simulink library "TorqueCommand"  (R2025a)
settings: Solver=VariableStepAuto  StartTime=0.0  StopTime=10.0  RelTol=1e-3
values from neighbouring files (symbols this model uses):
  RegenEnable : value not decoded    [TorqueCommand.sldd]
  TCEnable : value not decoded    [TorqueCommand.sldd]
undefined symbols (not defined in the file or in its folder): DiscIntNeverNeededParam, dt, raptor_xcp_function, TorqueKiLowerSat, TorqueKiUpperSat
libraries: Raptor_lib x56, Utilities x14, simulink x7, $bdroot x5
(part 1 of 2)
settings Model: Creator=serga  LastModifiedBy=hyuga

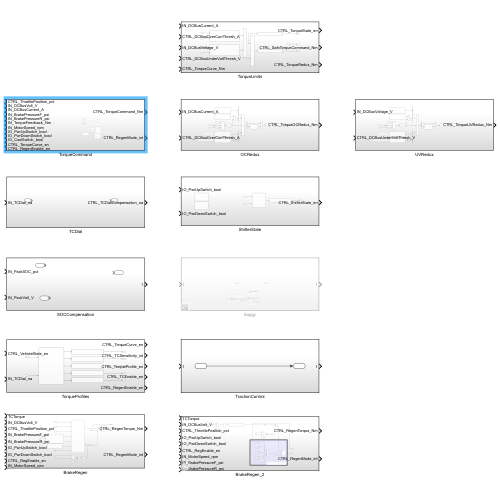
[thumbnail: Simulink's stored preview of the top-level diagram]
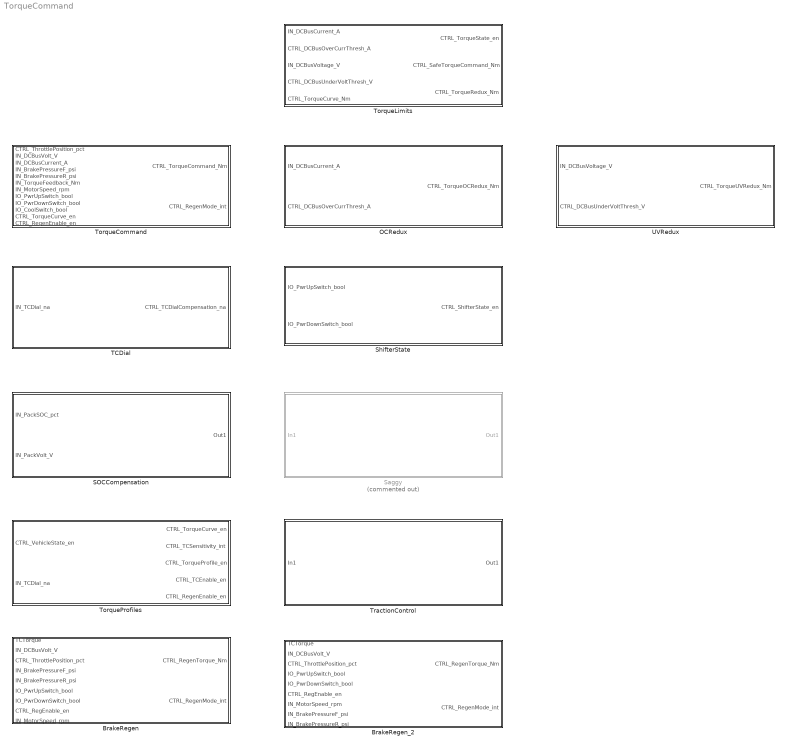
== system TorqueCommand ==
  BrakeRegen : Subsystem
  BrakeRegen_2 : Subsystem  AncestorBlock=TorqueCommand/BrakeRegen
  OCRedux : Subsystem
  SOCCompensation : Subsystem
  Saggy : Subsystem  Commented=on
  ShifterState : Subsystem
  TCDial : Subsystem
  TorqueCommand : Subsystem
  TorqueLimits : Subsystem
  TorqueProfiles : Subsystem
  TractionControl : Subsystem
  UVRedux : Subsystem

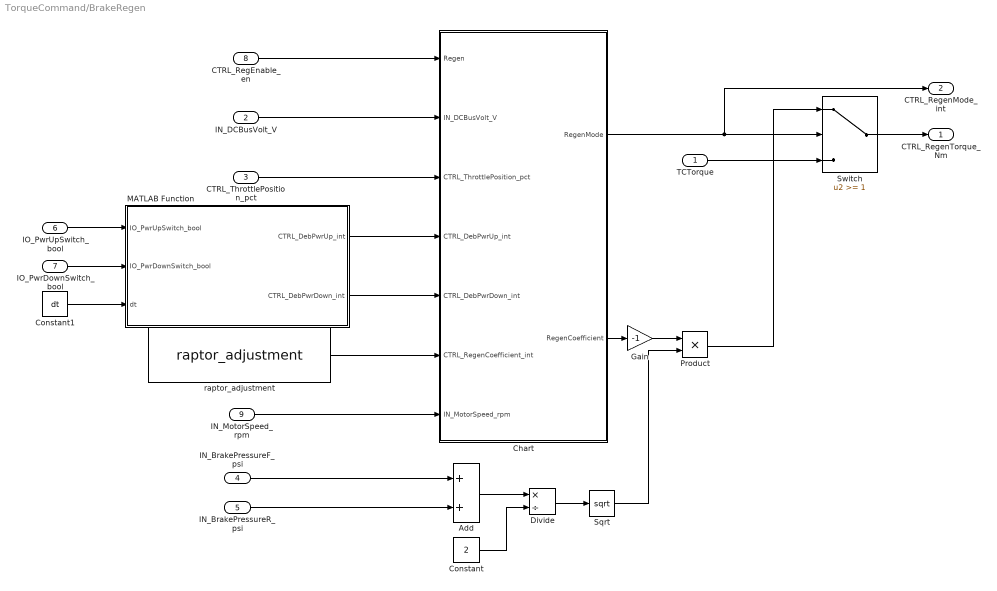
== system TorqueCommand/BrakeRegen ==
  TCTorque : Inport
  IN_DCBusVolt_V : Inport  Port=2
  CTRL_ThrottlePosition_pct : Inport  Port=3
  IN_BrakePressureF_psi : Inport  Port=4
  IN_BrakePressureR_psi : Inport  Port=5
  IO_PwrUpSwitch_bool : Inport  Port=6
  IO_PwrDownSwitch_bool : Inport  Port=7
  CTRL_RegEnable_en : Inport  Port=8
  IN_MotorSpeed_rpm : Inport  Port=9
  Add : Sum
  Chart : Stateflow chart  TreatAsAtomicUnit=on
  Constant : Constant  Value=2
  Constant1 : Constant  Value=dt
  Divide : Product  Inputs=*/
  Gain : Gain  Gain=-1
  MATLAB Function : MATLAB Function  TreatAsAtomicUnit=on
  Product : Product
  Sqrt : Sqrt
  Switch : Switch  Threshold=1  SaturateOnIntegerOverflow=off  InputSameDT=off
  raptor_adjustment : Raptor_lib/Data Storage/raptor_adjustment  paramName='CTRL_RegenCoefficient_int'  nameSource=Parameter  initValue=4  dataType=double  storage=Calibration  calDispType=Number  calEnum={'False', 'True'}  calGain=1.0  calOffset=0.0  calMax=inf  calMin=-inf  calFormat='-1'  calUnit=''  calHelp=''  calAccess=1  calFunction=raptor_xcp_function(gcb)  calDispHeaders=off  calColHeaders={'Col1' 'Col2' 'Col3'}  calRowHeaders={'Row1' 'Row2' 'Row3'}
      settings: SourceProductName=Raptor
  CTRL_RegenTorque_Nm : Outport
  CTRL_RegenMode_int : Outport  Port=2
  wires:
  Gain/1 -> Product/1
  Chart/2(RegenCoefficient) -> Gain/1
  IN_MotorSpeed_rpm/1 -> Chart/7(IN_MotorSpeed_rpm)
  Switch/1 -> CTRL_RegenTorque_Nm/1
  Product/1 -> Switch/1
  raptor_adjustment/1 -> Chart/6(CTRL_RegenCoefficient_int)
  TCTorque/1 -> Switch/3
  Sqrt/1 -> Product/2
  IN_DCBusVolt_V/1 -> Chart/2(IN_DCBusVolt_V)
  CTRL_ThrottlePosition_pct/1 -> Chart/3(CTRL_ThrottlePosition_pct)
  Add/1 -> Divide/1
  Constant/1 -> Divide/2
  IN_BrakePressureF_psi/1 -> Add/1
  IN_BrakePressureR_psi/1 -> Add/2
  Divide/1 -> Sqrt/1
  Chart/1(RegenMode) -> Switch/2, CTRL_RegenMode_int/1
  Constant1/1 -> MATLAB Function/3(dt)
  IO_PwrDownSwitch_bool/1 -> MATLAB Function/2(IO_PwrDownSwitch_bool)
  IO_PwrUpSwitch_bool/1 -> MATLAB Function/1(IO_PwrUpSwitch_bool)
  MATLAB Function/1(CTRL_DebPwrUp_int) -> Chart/4(CTRL_DebPwrUp_int)
  MATLAB Function/2(CTRL_DebPwrDown_int) -> Chart/5(CTRL_DebPwrDown_int)
  CTRL_RegEnable_en/1 -> Chart/1(Regen)

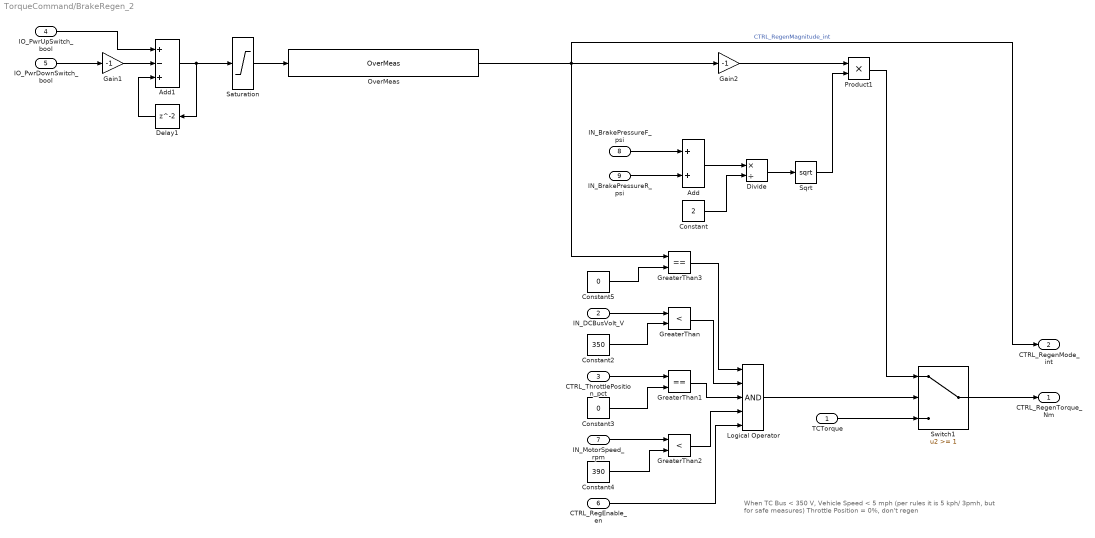
== system TorqueCommand/BrakeRegen_2 ==
  note: When TC Bus < 350 V,
      | Vehicle Speed < 5 mph (per rules it is 5 kph/ 3pmh, but for safe measures)
      | Throttle Position = 0%,
      | don't regen
  TCTorque : Inport
  IN_DCBusVolt_V : Inport  Port=2
  CTRL_ThrottlePosition_pct : Inport  Port=3
  IO_PwrUpSwitch_bool : Inport  Port=4
  IO_PwrDownSwitch_bool : Inport  Port=5
  CTRL_RegEnable_en : Inport  Port=6
  IN_MotorSpeed_rpm : Inport  Port=7
  IN_BrakePressureF_psi : Inport  Port=8
  IN_BrakePressureR_psi : Inport  Port=9
  Add : Sum
  Add1 : Sum  Inputs=+-+
  Constant : Constant  Value=2
  Constant2 : Constant  Value=350
  Constant3 : Constant  Value=0
  Constant4 : Constant  Value=390
  Constant5 : Constant  Value=0
  Delay1 : Delay
  Divide : Product  Inputs=*/
  Gain1 : Gain  Gain=-1
  Gain2 : Gain  Gain=-1
  GreaterThan : RelationalOperator  Operator=<  OutDataTypeStr=boolean  RndMeth=Simplest  InputSameDT=off
  GreaterThan1 : RelationalOperator  Operator===  OutDataTypeStr=boolean  RndMeth=Simplest  InputSameDT=off
  GreaterThan2 : RelationalOperator  Operator=<  OutDataTypeStr=boolean  RndMeth=Simplest  InputSameDT=off
  GreaterThan3 : RelationalOperator  Operator===  OutDataTypeStr=boolean  RndMeth=Simplest  InputSameDT=off
  Logical Operator : Logic  Inputs=5  AllPortsSameDT=off  OutDataTypeStr=boolean
  OverMeas : Utilities/OverMeas  sigName='CTRL_RegenMagnitude_int'  minimum=0  maximum=7
  Product1 : Product
  Saturation : Saturate  UpperLimit=7  LowerLimit=0
  Sqrt : Sqrt
  Switch1 : Switch  Threshold=1  SaturateOnIntegerOverflow=off  InputSameDT=off
  CTRL_RegenTorque_Nm : Outport
  CTRL_RegenMode_int : Outport  Port=2
  wires:
  Switch1/1 -> CTRL_RegenTorque_Nm/1
  Product1/1 -> Switch1/1
  Gain2/1 -> Product1/1
  IN_BrakePressureR_psi/1 -> Add/2
  Constant/1 -> Divide/2
  Add/1 -> Divide/1
  IN_BrakePressureF_psi/1 -> Add/1
  Divide/1 -> Sqrt/1
  Sqrt/1 -> Product1/2
  CTRL_RegEnable_en/1 -> Logical Operator/5
  GreaterThan2/1 -> Logical Operator/4
  GreaterThan1/1 -> Logical Operator/3
  GreaterThan/1 -> Logical Operator/2
  GreaterThan3/1 -> Logical Operator/1
  Constant5/1 -> GreaterThan3/2
  OverMeas/1 -> GreaterThan3/1, CTRL_RegenMode_int/1, Gain2/1  "CTRL_RegenMagnitude_int"
  TCTorque/1 -> Switch1/3
  Saturation/1 -> OverMeas/1
  Delay1/1 -> Add1/3
  Add1/1 -> Delay1/1, Saturation/1
  Gain1/1 -> Add1/2
  IO_PwrUpSwitch_bool/1 -> Add1/1
  IO_PwrDownSwitch_bool/1 -> Gain1/1
  Logical Operator/1 -> Switch1/2
  Constant4/1 -> GreaterThan2/2
  IN_MotorSpeed_rpm/1 -> GreaterThan2/1
  Constant3/1 -> GreaterThan1/2
  CTRL_ThrottlePosition_pct/1 -> GreaterThan1/1
  IN_DCBusVolt_V/1 -> GreaterThan/1
  Constant2/1 -> GreaterThan/2

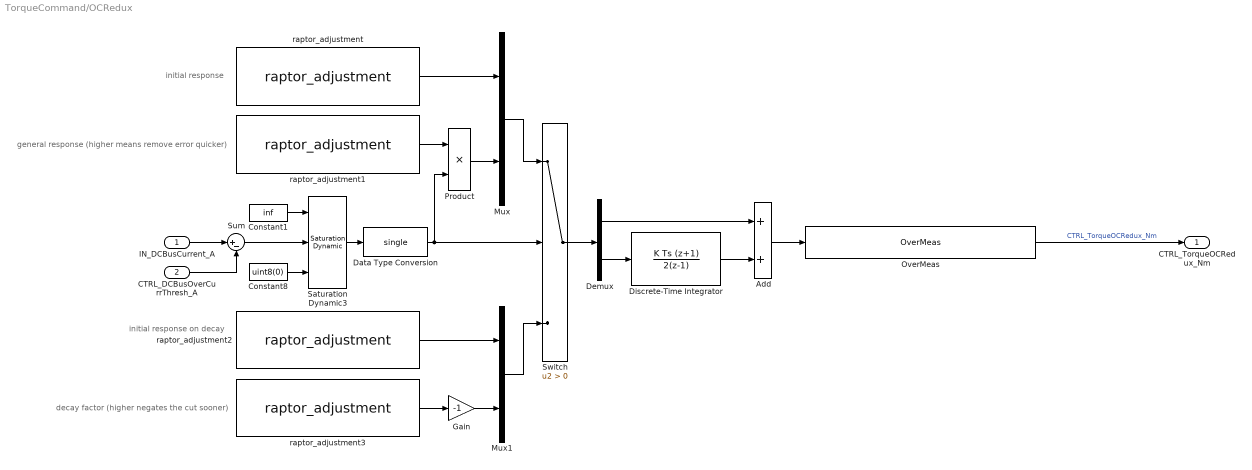
== system TorqueCommand/OCRedux ==
  note: general response (higher means remove error quicker)
  note: initial response
  note: initial response on decay
  note: decay factor (higher negates the cut sooner)
  IN_DCBusCurrent_A : Inport
  CTRL_DCBusOverCurrThresh_A : Inport  Port=2
  Add : Sum
  Constant1 : Constant  Value=inf
  Constant8 : Constant  Value=uint8(0)
  Data Type Conversion : DataTypeConversion  OutDataTypeStr=single  SaturateOnIntegerOverflow=off  RndMeth=Floor
  Demux : Demux  Outputs=2
  Discrete-Time Integrator : DiscreteIntegrator  IntegratorMethod=Integration: Trapezoidal  SampleTime=-1  LimitOutput=on  UpperSaturationLimit=TorqueKiUpperSat  LowerSaturationLimit=TorqueKiLowerSat  ICPrevOutput=DiscIntNeverNeededParam  ICPrevScaledInput=DiscIntNeverNeededParam
  Gain : Gain  Gain=-1
  Mux : Mux  Inputs=2
  Mux1 : Mux  Inputs=2
  OverMeas : Utilities/OverMeas  sigName='CTRL_TorqueOCRedux_Nm'  minimum=-inf  maximum=inf
  Product : Product
  Saturation Dynamic3 : simulink/Discontinuities/Saturation Dynamic  OutMin=[]  OutMax=[]  OutDataTypeStr=Inherit: Same as second input  OutDataType=fixdt(1, 16)  OutScaling=2^-10  DoSatur=off
  Sum : Sum  Inputs=|+-
  Switch : Switch  Criteria=u2 > Threshold  SaturateOnIntegerOverflow=off  InputSameDT=off
  raptor_adjustment : Raptor_lib/Data Storage/raptor_adjustment  paramName='CTRL_CurrKpLim_na'  nameSource=Parameter  initValue=10  dataType=single  storage=Calibration  calDispType=Number  calEnum={'False', 'True'}  calGain=1.0  calOffset=0.0  calMax=inf  calMin=-inf  calFormat='-1'  calUnit=''  calHelp=''  calAccess=1  calFunction=raptor_xcp_function(gcb)  calDispHeaders=off  calColHeaders={'Col1' 'Col2' 'Col3'}  calRowHeaders={'Row1' 'Row2' 'Row3'}
      settings: SourceProductName=Raptor
  raptor_adjustment1 : Raptor_lib/Data Storage/raptor_adjustment  paramName='CTRL_CurrKiLim_na'  nameSource=Parameter  initValue=2  dataType=single  storage=Calibration  calDispType=Number  calEnum={'False', 'True'}  calGain=1.0  calOffset=0.0  calMax=inf  calMin=-inf  calFormat='-1'  calUnit=''  calHelp=''  calAccess=1  calFunction=raptor_xcp_function(gcb)  calDispHeaders=off  calColHeaders={'Col1' 'Col2' 'Col3'}  calRowHeaders={'Row1' 'Row2' 'Row3'}
      settings: SourceProductName=Raptor
  raptor_adjustment2 : Raptor_lib/Data Storage/raptor_adjustment  paramName='CTRL_CurrKpLimDecay_na'  nameSource=Parameter  initValue=0  dataType=single  storage=Calibration  calDispType=Number  calEnum={'False', 'True'}  calGain=1.0  calOffset=0.0  calMax=inf  calMin=-inf  calFormat='-1'  calUnit=''  calHelp=''  calAccess=1  calFunction=raptor_xcp_function(gcb)  calDispHeaders=off  calColHeaders={'Col1' 'Col2' 'Col3'}  calRowHeaders={'Row1' 'Row2' 'Row3'}
      settings: SourceProductName=Raptor
  raptor_adjustment3 : Raptor_lib/Data Storage/raptor_adjustment  paramName='CTRL_CurrKiLimDecay_na'  nameSource=Parameter  initValue=250  dataType=single  storage=Calibration  calDispType=Number  calEnum={'False', 'True'}  calGain=1.0  calOffset=0.0  calMax=inf  calMin=-inf  calFormat='-1'  calUnit=''  calHelp=''  calAccess=1  calFunction=raptor_xcp_function(gcb)  calDispHeaders=off  calColHeaders={'Col1' 'Col2' 'Col3'}  calRowHeaders={'Row1' 'Row2' 'Row3'}
      settings: SourceProductName=Raptor
  CTRL_TorqueOCRedux_Nm : Outport
  wires:
  Saturation Dynamic3/1 -> Data Type Conversion/1
  Discrete-Time Integrator/1 -> Add/2
  Demux/2 -> Discrete-Time Integrator/1
  Constant8/1 -> Saturation Dynamic3/3
  Constant1/1 -> Saturation Dynamic3/1
  Data Type Conversion/1 -> Switch/2, Product/2
  Sum/1 -> Saturation Dynamic3/2
  CTRL_DCBusOverCurrThresh_A/1 -> Sum/2
  IN_DCBusCurrent_A/1 -> Sum/1
  OverMeas/1 -> CTRL_TorqueOCRedux_Nm/1  "CTRL_TorqueOCRedux_Nm"
  Add/1 -> OverMeas/1
  Demux/1 -> Add/1
  Switch/1 -> Demux/1
  Mux1/1 -> Switch/3
  raptor_adjustment2/1 -> Mux1/1
  Gain/1 -> Mux1/2
  raptor_adjustment3/1 -> Gain/1
  Mux/1 -> Switch/1
  raptor_adjustment/1 -> Mux/1
  Product/1 -> Mux/2
  raptor_adjustment1/1 -> Product/1

== system TorqueCommand/SOCCompensation ==
  IN_PackSOC_pct : Inport
  IN_PackVolt_V : Inport  Port=2
  Out1 : Outport

== system TorqueCommand/Saggy ==
  note: motor speed
  note: angular acceleration (rad/s)
  note: torque feedback (net torque)
  note: force of motor
  note: want to detect voltage sag before it happens
  note: maximize torque while reducing current draw
  note: motor mechanical power
  In1 : Inport
  Demux : Demux  Outputs=2
  Display : Display
  Divide1 : Product  Commented=on  Inputs=*/
  From Workspace : FromWorkspace  VariableName=imu_input  SampleTime=-1
  Gain : Gain  Gain=(2*pi)/60
  Ground : Ground
  Product : Product
  Scope : Scope
  Terminator : Terminator
  raptor_adjustment2 : Raptor_lib/Data Storage/raptor_adjustment  Commented=on  paramName='CTRL_MotorIntertia_kgm2'  nameSource=Parameter  initValue=0.0383  dataType=double  storage=Calibration  calDispType=Number  calEnum={'False', 'True'}  calGain=1.0  calOffset=0.0  calMax=inf  calMin=-inf  calFormat='-1'  calUnit=''  calHelp=''  calAccess=1  calFunction=raptor_xcp_function(gcb)  calDispHeaders=off  calColHeaders={'Col1' 'Col2' 'Col3'}  calRowHeaders={'Row1' 'Row2' 'Row3'}
      settings: SourceProductName=Raptor
  Out1 : Outport
  wires:
  In1/1 -> Terminator/1
  Ground/1 -> Out1/1
  raptor_adjustment2/1 -> Divide1/2
  Divide1/1 -> ?
  Gain/1 -> Product/2
  From Workspace/1 -> Demux/1
  Demux/1 -> Product/1
  Demux/2 -> Gain/1
  Product/1 -> Display/1, Scope/1

== system TorqueCommand/ShifterState ==
  IO_PwrUpSwitch_bool : Inport
  IO_PwrDownSwitch_bool : Inport  Port=2
  EnumeratedOverMeas : Utilities/EnumeratedOverMeas  sigName='CTRL_ShifterState_en'  enumName='TorqueState'
  MATLAB Function : MATLAB Function  TreatAsAtomicUnit=on
  Subsystem : Subsystem  Commented=on
  Subsystem1 : Subsystem  Commented=on
  CTRL_ShifterState_en : Outport
  wires:
  EnumeratedOverMeas/1 -> CTRL_ShifterState_en/1  "CTRL_ShifterState_en"
  MATLAB Function/1(stateNum) -> EnumeratedOverMeas/1
  IO_PwrDownSwitch_bool/1 -> MATLAB Function/2(IO_PwrDownSwitch_bool)
  IO_PwrUpSwitch_bool/1 -> MATLAB Function/1(IO_PwrUpSwitch_bool)

== system TorqueCommand/TCDial ==
  IN_TCDial_na : Inport
  CTRL_TCDialCompensation_na : Outport

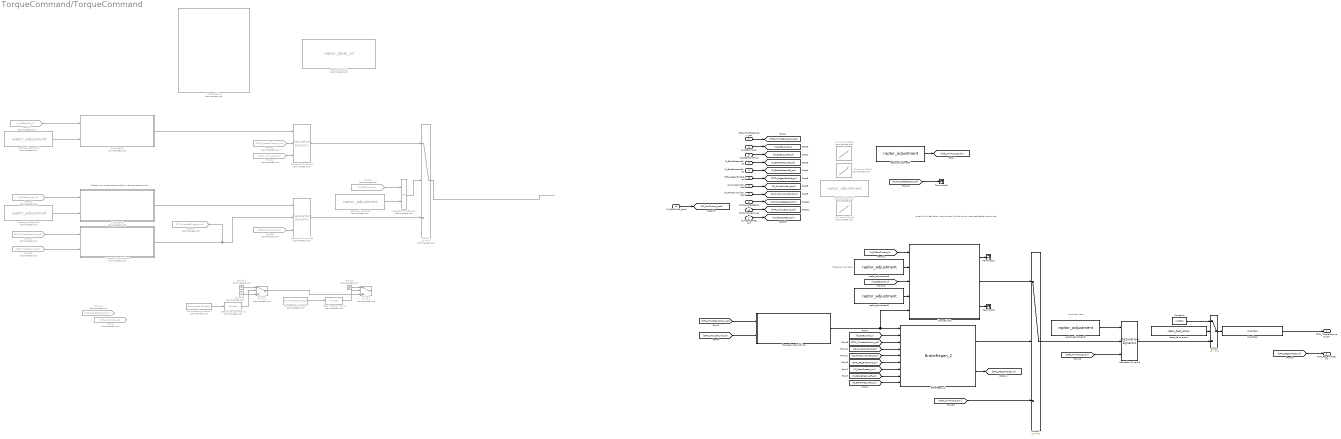
== system TorqueCommand/TorqueCommand ==
  note: these are hard caps
  note: if there is an overcurrent condition, set new torque limit
  note: hard cap here
  note: current limit (set below legit current limit to have more predictable torque loss)
  CTRL_ThrottlePosition_pct : Inport
  IN_DCBusVolt_V : Inport  Port=2
  IN_DCBusCurrent_A : Inport  Port=3
  IN_BrakePressureF_psi : Inport  Port=4
  IN_BrakePressureR_psi : Inport  Port=5
  IN_TorqueFeedback_Nm : Inport  Port=6
  IN_MotorSpeed_rpm : Inport  Port=7
  IO_PwrUpSwitch_bool : Inport  Port=8
  IO_PwrDownSwitch_bool : Inport  Port=9
  IO_CoolSwitch_bool : Inport  Port=10
  CTRL_TorqueCurve_en : Inport  Port=11
  CTRL_RegenEnable_en : Inport  Port=12
  1-D Lookup Table : Lookup_n-D  Commented=on  NumberOfTableDimensions=1  BreakpointsForDimension1=[0;50;100;120;130;140;150;160;170;180;190;200;205;210;215;220;225;230;235;240;245;250;255;260;265;270;275;280;285;290;295;300]  Table=[200;200;200;200;200;200;200;200;200;200;200;200;200;200;200;200;200;200;200;200;200;200;195;190;185;180;175;170;165;160;155;150]  InternalRulePriority=Speed  RndMeth=Simplest
  1-D Lookup Table1 : Lookup_n-D  Commented=on  NumberOfTableDimensions=1  BreakpointsForDimension1=[0;5;10;15;20;25;30;35;40;45;50;55;60;65;70;75;80;85;90;95;100]  Table=[0;3;6;9;12;15;25;35;45;55;65;75;85;95;105;115;135;155;175;195;200]  InternalRulePriority=Speed  RndMeth=Simplest
  1-D Lookup Table2 : Lookup_n-D  Commented=on  NumberOfTableDimensions=1  BreakpointsForDimension1=[0;100;200;205;210;215;220;225;230;235;240;245;250;255;260;265;270;275;280;285;290;300;310;320;330;400]  Table=[0;0;0;25;50;100;125;150;155;160;165;170;175;180;185;190;192;194;196;198;200;200;200;200;200;200]  InternalRulePriority=Speed  RndMeth=Simplest
  BrakeRegen_2 : $bdroot/BrakeRegen_2  SystemSampleTime=-1  VariantActivationTime=update diagram  EmptyChoice=off  PassThrough=off  PassThroughVariantControl=(default)  EmptyChoiceVariantControl=(default)  AllowFlexibleInterface=on  Latency=0  AutoFrameSizeCalculation=off
  Constant1 : Constant  Value=uint8(0)
  Data Type Conversion : DataTypeConversion  Commented=on  OutDataTypeStr=boolean  SaturateOnIntegerOverflow=off  RndMeth=Floor
  Data Type Conversion1 : DataTypeConversion  Commented=on  OutDataTypeStr=boolean  SaturateOnIntegerOverflow=off  RndMeth=Floor
  Enumerated Constant : simulink/Sources/Enumerated Constant  Commented=on  OutDataTypeStr=Enum: RegenEnable  Value=RegenEnable.On  SampleTime=inf
  Enumerated Constant1 : simulink/Sources/Enumerated Constant  Commented=on  OutDataTypeStr=Enum: TCEnable  Value=TCEnable.On  SampleTime=inf
  From16 : From  Commented=on  GotoTag=IN_TorqueFeedback_Nm
  From23 : From  Commented=on  GotoTag=IN_DCBusVolt_V
  From24 : From  Commented=on  GotoTag=IN_DCBusVolt_V
  From25 : From  Commented=on  GotoTag=CTRL_AssistedTorque_Nm
  From26 : From  Commented=on  GotoTag=CTRL_MinTorque_Nm
  From27 : From  Commented=on  GotoTag=CTRL_ThrottlePosition_pct
  From28 : From  Commented=on  GotoTag=CTRL_MinTorque_Nm
  From29 : From  Commented=on  GotoTag=CTRL_TorqueCurve_en
  From30 : From  Commented=on  GotoTag=IN_DCBusCurrent_A
  From6 : From  Commented=on  GotoTag=CTRL_SlipRatio_na
  Goto14 : Goto  Commented=on  GotoTag=CTRL_AssistedTorque_Nm
  GreaterThanOrEqual2 : RelationalOperator  Commented=on  Operator=<=  OutDataTypeStr=boolean  RndMeth=Simplest  InputSameDT=off
  Ground : Ground  Commented=on
  Ground1 : Ground  Commented=on
  Ground2 : Ground  Commented=on
  OverMeas : Utilities/OverMeas  sigName='CTRL_TorqueCommand_Nm'  minimum=0  maximum=240
  Saturation Dynamic : simulink/Discontinuities/Saturation Dynamic  OutMin=[]  OutMax=[]  OutDataTypeStr=Inherit: Same as second input  OutDataType=fixdt(1, 16)  OutScaling=2^-10  DoSatur=off
  Saturation Dynamic3 : simulink/Discontinuities/Saturation Dynamic  Commented=on  OutMin=[]  OutMax=[]  OutDataTypeStr=Inherit: Same as second input  OutDataType=fixdt(1, 16)  OutScaling=2^-10  DoSatur=off
  Saturation Dynamic4 : simulink/Discontinuities/Saturation Dynamic  Commented=on  OutMin=[]  OutMax=[]  OutDataTypeStr=Inherit: Same as second input  OutDataType=fixdt(1, 16)  OutScaling=2^-10  DoSatur=off
  Subsystem2 : Subsystem  Commented=on
  Subsystem3 : Subsystem  Commented=on
  Switch : Switch  Criteria=u2 ~= 0  SaturateOnIntegerOverflow=off  InputSameDT=off
  Switch1 : Switch  Commented=on  Criteria=u2 ~= 0  OutDataTypeStr=single  SaturateOnIntegerOverflow=off  InputSameDT=off
  Switch2 : Switch  Criteria=u2 ~= 0  OutDataTypeStr=single  SaturateOnIntegerOverflow=off  InputSameDT=off
  Switch4 : Switch  Commented=on  Criteria=u2 ~= 0  SaturateOnIntegerOverflow=off  InputSameDT=off
  Switch5 : Switch  Commented=on  Criteria=u2 ~= 0  SaturateOnIntegerOverflow=off  InputSameDT=off
  Terminator1 : Terminator
  Terminator2 : Terminator
  Terminator3 : Terminator
  TorqueCeiling : Stateflow chart  Commented=on  TreatAsAtomicUnit=on
  TorqueCurveSwitching : Subsystem
  TorqueCurveSwitching1 : Subsystem  Commented=on
  TorqueLimits : Subsystem  AncestorBlock=TorqueCommand/TorqueLimits
  raptor_adjustment1 : Raptor_lib/Data Storage/raptor_adjustment  paramName='CTRL_DCBusUnderVoltThresh_V'  nameSource=Parameter  initValue=250  dataType=single  storage=Calibration  calDispType=Number  calEnum={'False', 'True'}  calGain=1.0  calOffset=0.0  calMax=378  calMin=-inf  calFormat='-1'  calUnit=''  calHelp=''  calAccess=1  calFunction=raptor_xcp_function(gcb)  calDispHeaders=off  calColHeaders={'Col1' 'Col2' 'Col3'}  calRowHeaders={'Row1' 'Row2' 'Row3'}
      settings: SourceProductName=Raptor
  raptor_adjustment10 : Raptor_lib/Data Storage/raptor_adjustment  Commented=on  paramName='CTRL_CurrentTorqueLimitSetting_na'  nameSource=Parameter  initValue=1  dataType=double  storage=Calibration  calDispType=Number  calEnum={'False', 'True'}  calGain=1.0  calOffset=0.0  calMax=3  calMin=1  calFormat='-1'  calUnit=''  calHelp=''  calAccess=1  calFunction=raptor_xcp_function(gcb)  calDispHeaders=off  calColHeaders={'Col1' 'Col2' 'Col3'}  calRowHeaders={'Row1' 'Row2' 'Row3'}
      settings: SourceProductName=Raptor
  raptor_adjustment11 : Raptor_lib/Data Storage/raptor_adjustment  Commented=on  paramName='CTRL_VoltageTorqueLimitSetting_Nm'  nameSource=Parameter  initValue=1  dataType=double  storage=Calibration  calDispType=Number  calEnum={'False', 'True'}  calGain=1.0  calOffset=0.0  calMax=3  calMin=1  calFormat='-1'  calUnit=''  calHelp=''  calAccess=1  calFunction=raptor_xcp_function(gcb)  calDispHeaders=off  calColHeaders={'Col1' 'Col2' 'Col3'}  calRowHeaders={'Row1' 'Row2' 'Row3'}
      settings: SourceProductName=Raptor
  raptor_adjustment2 : Raptor_lib/Data Storage/raptor_adjustment  paramName='CTRL_MaxTorque'  nameSource=Parameter  initValue=200  dataType=single  storage=Calibration  calDispType=Number  calEnum={'False', 'True'}  calGain=1.0  calOffset=0.0  calMax=230  calMin=0  calFormat='-1'  calUnit=''  calHelp=''  calAccess=1  calFunction=raptor_xcp_function(gcb)  calDispHeaders=off  calColHeaders={'Col1' 'Col2' 'Col3'}  calRowHeaders={'Row1' 'Row2' 'Row3'}
      settings: SourceProductName=Raptor
  raptor_adjustment3 : Raptor_lib/Data Storage/raptor_adjustment  Commented=on  paramName='CTRL_TorqueCurrLim_Nm'  nameSource=Parameter  initValue=100  dataType=single  storage=Calibration  calDispType=Number  calEnum={'False', 'True'}  calGain=1.0  calOffset=0.0  calMax=inf  calMin=-inf  calFormat='-1'  calUnit=''  calHelp=''  calAccess=1  calFunction=raptor_xcp_function(gcb)  calDispHeaders=off  calColHeaders={'Col1' 'Col2' 'Col3'}  calRowHeaders={'Row1' 'Row2' 'Row3'}
      settings: SourceProductName=Raptor
  raptor_adjustment5 : Raptor_lib/Data Storage/raptor_adjustment  paramName='CTRL_MinTorque'  nameSource=Parameter  initValue=-50  dataType=single  storage=Calibration  calDispType=Number  calEnum={'False', 'True'}  calGain=1.0  calOffset=0.0  calMax=230  calMin=-250  calFormat='-1'  calUnit=''  calHelp=''  calAccess=1  calFunction=raptor_xcp_function(gcb)  calDispHeaders=off  calColHeaders={'Col1' 'Col2' 'Col3'}  calRowHeaders={'Row1' 'Row2' 'Row3'}
      settings: SourceProductName=Raptor
  raptor_adjustment8 : Raptor_lib/Data Storage/raptor_adjustment  paramName='CTRL_DCBusOverCurrThresh_A'  nameSource=Parameter  initValue=140  dataType=single  storage=Calibration  calDispType=Number  calEnum={'False', 'True'}  calGain=1.0  calOffset=0.0  calMax=240  calMin=-inf  calFormat='-1'  calUnit=''  calHelp=''  calAccess=1  calFunction=raptor_xcp_function(gcb)  calDispHeaders=off  calColHeaders={'Col1' 'Col2' 'Col3'}  calRowHeaders={'Row1' 'Row2' 'Row3'}
      settings: SourceProductName=Raptor
  raptor_adjustment9 : Raptor_lib/Data Storage/raptor_adjustment  Commented=on  paramName='CTRL_DCBusUnderVoltThresh_V'  nameSource=Parameter  initValue=250  dataType=single  storage=Calibration  calDispType=Number  calEnum={'False', 'True'}  calGain=1.0  calOffset=0.0  calMax=240  calMin=-inf  calFormat='-1'  calUnit=''  calHelp=''  calAccess=1  calFunction=raptor_xcp_function(gcb)  calDispHeaders=off  calColHeaders={'Col1' 'Col2' 'Col3'}  calRowHeaders={'Row1' 'Row2' 'Row3'}
      settings: SourceProductName=Raptor
  raptor_fault_action : Raptor_lib/Faults/raptor_fault_action  actionName='TorqueCmdOverride'  calVisible=on  calAccess=1  calFunction='System | FaultManager | FaultAction'
      settings: SourceProductName=Raptor
  raptor_table_1d3 : Raptor_lib/Table Lookup/raptor_table_1d  Commented=on  dataName='CTRL_TargetSlipRatio_1D'  initValue=[0;764;1528;2293;3057;3822;4586;5350;6114;6880;7643]  dataType=single  storage=Calibration  initValueX=[12;12;12;12;12;12;11.5;11;10.5;10;8]  dataTypeXY=single  storageXY=Calibration  calVisible=on  showTable=on  calGain=1.0  calOffset=0.0  calMax=Inf  calMin=-Inf  calFormat='-1'  calUnit='pct'  calHelp=''  showBreakpoint=on  dataNameX=[]  calGainX=1.0  calOffsetX=0.0  calMaxX=Inf  calMinX=-Inf  calFormatX='-1'  calUnitX='rpm'  calHelpX=''  calAccess=1  calFunction=raptor_xcp_function(gcb)  measureEnable=off  mName=['Data1D_Output']
      settings: SourceProductName=Raptor
  CTRL_TorqueCommand_Nm : Outport
  CTRL_RegenMode_int : Outport  Port=2
  wires:
  [IN_BrakePressureR_psi] -> BrakeRegen_2/9
  [IN_BrakePressureF_psi] -> BrakeRegen_2/8
  [IN_MotorSpeed_rpm] -> BrakeRegen_2/7
  [CTRL_RegenEnable_en] -> BrakeRegen_2/6
  [IO_PwrDownSwitch_bool] -> BrakeRegen_2/5
  [IO_PwrUpSwitch_bool] -> BrakeRegen_2/4
  [IN_DCBusVolt_V] -> BrakeRegen_2/2
  [CTRL_ThrottlePosition_pct] -> BrakeRegen_2/3
  BrakeRegen_2/1 -> Switch2/2
  IN_MotorSpeed_rpm/1 -> [IN_MotorSpeed_rpm]
  [IN_TorqueFeedback_Nm] -> Terminator3/1
  [CTRL_RegenMode_int] -> CTRL_RegenMode_int/1
  BrakeRegen_2/2 -> [CTRL_RegenMode_int]
  TorqueLimits/3(CTRL_TorqueRedux_Nm) -> Terminator2/1
  Constant1/1 -> Switch/1
  Switch/1 -> OverMeas/1
  OverMeas/1 -> CTRL_TorqueCommand_Nm/1  "CTRL_TorqueCommand_Nm"
  raptor_fault_action/1 -> Switch/2
  Saturation Dynamic/1 -> Switch/3
  Switch2/1 -> Saturation Dynamic/2
  [CTRL_ThrottlePosition_pct] -> TorqueCurveSwitching/1(CTRL_ThrottlePosition_pct)
  IN_DCBusVolt_V/1 -> [IN_DCBusVolt_V]
  IN_DCBusCurrent_A/1 -> [IN_DCBusCurrent_A]
  CTRL_ThrottlePosition_pct/1 -> [CTRL_ThrottlePosition_pct]
  IN_BrakePressureF_psi/1 -> [IN_BrakePressureF_psi]
  IN_BrakePressureR_psi/1 -> [IN_BrakePressureR_psi]
  CTRL_RegenEnable_en/1 -> [CTRL_RegenEnable_en]
  [CTRL_TorqueCurve_en] -> TorqueCurveSwitching/2(CTRL_TorqueCurve_en)
  IO_PwrDownSwitch_bool/1 -> [IO_PwrDownSwitch_bool]
  IO_PwrUpSwitch_bool/1 -> [IO_PwrUpSwitch_bool]
  IN_TorqueFeedback_Nm/1 -> [IN_TorqueFeedback_Nm]
  Ground/1 -> Switch4/1
  Switch5/1 -> Switch4/3
  Enumerated Constant/1 -> Data Type Conversion/1
  Enumerated Constant1/1 -> Data Type Conversion1/1
  Data Type Conversion/1 -> Switch4/2
  Data Type Conversion1/1 -> Switch5/2
  Ground1/1 -> Switch5/1
  Ground2/1 -> Switch5/3
  raptor_adjustment5/1 -> [CTRL_MinTorque_Nm]
  [CTRL_MinTorque_Nm] -> Saturation Dynamic/3
  CTRL_TorqueCurve_en/1 -> [CTRL_TorqueCurve_en]
  IO_CoolSwitch_bool/1 -> [IO_CoolSwitch_bool]
  [IN_DCBusCurrent_A] -> TorqueLimits/1(IN_DCBusCurrent_A)
  raptor_adjustment1/1 -> TorqueLimits/4(CTRL_DCBusUnderVoltThresh_V)
  raptor_adjustment8/1 -> TorqueLimits/2(CTRL_DCBusOverCurrThresh_A)
  TorqueCurveSwitching1/1(Torque) -> Saturation Dynamic3/2, Goto14/1
  raptor_adjustment11/1 -> Subsystem3/2(CTRL_VoltageTorqueSetting_na)
  raptor_adjustment10/1 -> Subsystem2/2(CTRL_CurrentTorqueSetting_na)
  From28/1 -> Saturation Dynamic3/3
  From26/1 -> Saturation Dynamic4/3
  From25/1 -> Saturation Dynamic4/2
  From23/1 -> GreaterThanOrEqual2/1
  From30/1 -> Subsystem2/1(IN_DCBusCurrent_A)
  From29/1 -> TorqueCurveSwitching1/2(CTRL_TorqueCurve_en)
  From27/1 -> TorqueCurveSwitching1/1(CTRL_ThrottlePosition_pct)
  Switch1/1 -> ?
  raptor_adjustment9/1 -> GreaterThanOrEqual2/2
  GreaterThanOrEqual2/1 -> Switch1/2
  Saturation Dynamic4/1 -> Switch1/1
  Subsystem3/1(CTRL_CurrentTorqueLimit_Nm) -> Saturation Dynamic4/1
  From24/1 -> Subsystem3/1(IN_DCBusVoltage_V)
  Subsystem2/1(CTRL_CurrentTorqueLimit_Nm) -> Saturation Dynamic3/1
  Saturation Dynamic3/1 -> Switch1/3
  [CTRL_MinTorque_Nm] -> Switch2/3
  TorqueLimits/2(CTRL_SafeTorqueCommand_Nm) -> Switch2/1
  raptor_adjustment2/1 -> Saturation Dynamic/1
  TorqueCurveSwitching/1(Torque) -> TorqueLimits/5(CTRL_TorqueCurve_Nm), BrakeRegen_2/1
  [IN_DCBusVolt_V] -> TorqueLimits/3(IN_DCBusVoltage_V)
  TorqueLimits/1(CTRL_TorqueState_en) -> Terminator1/1

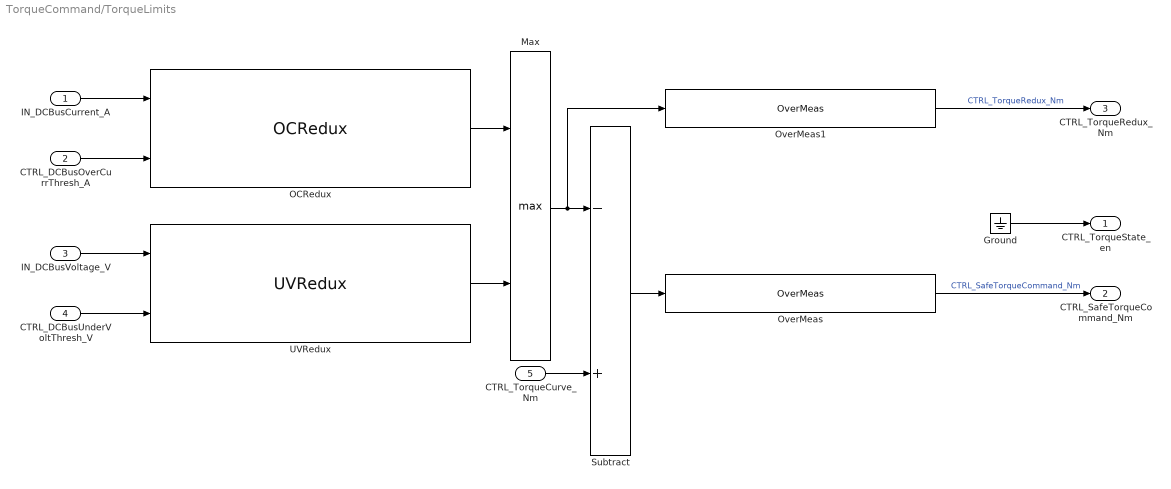
== system TorqueCommand/TorqueLimits ==
  IN_DCBusCurrent_A : Inport
  CTRL_DCBusOverCurrThresh_A : Inport  Port=2
  IN_DCBusVoltage_V : Inport  Port=3
  CTRL_DCBusUnderVoltThresh_V : Inport  Port=4
  CTRL_TorqueCurve_Nm : Inport  Port=5
  Ground : Ground
  Max : MinMax  Function=max  Inputs=2
  OCRedux : $bdroot/OCRedux  SystemSampleTime=-1  VariantActivationTime=update diagram  EmptyChoice=off  PassThrough=off  PassThroughVariantControl=(default)  EmptyChoiceVariantControl=(default)  AllowFlexibleInterface=on  Latency=0  AutoFrameSizeCalculation=off
  OverMeas : Utilities/OverMeas  sigName='CTRL_SafeTorqueCommand_Nm'  minimum=-inf  maximum=inf
  OverMeas1 : Utilities/OverMeas  sigName='CTRL_TorqueRedux_Nm'  minimum=-inf  maximum=inf
  Subtract : Sum  Inputs=-+
  UVRedux : $bdroot/UVRedux  SystemSampleTime=-1  VariantActivationTime=update diagram  EmptyChoice=off  PassThrough=off  PassThroughVariantControl=(default)  EmptyChoiceVariantControl=(default)  AllowFlexibleInterface=on  Latency=0  AutoFrameSizeCalculation=off
  CTRL_TorqueState_en : Outport
  CTRL_SafeTorqueCommand_Nm : Outport  Port=2
  CTRL_TorqueRedux_Nm : Outport  Port=3
  wires:
  OverMeas1/1 -> CTRL_TorqueRedux_Nm/1  "CTRL_TorqueRedux_Nm"
  Ground/1 -> CTRL_TorqueState_en/1
  CTRL_DCBusUnderVoltThresh_V/1 -> UVRedux/2
  IN_DCBusVoltage_V/1 -> UVRedux/1
  UVRedux/1 -> Max/2
  OverMeas/1 -> CTRL_SafeTorqueCommand_Nm/1  "CTRL_SafeTorqueCommand_Nm"
  Subtract/1 -> OverMeas/1
  CTRL_TorqueCurve_Nm/1 -> Subtract/2
  Max/1 -> Subtract/1, OverMeas1/1
  CTRL_DCBusOverCurrThresh_A/1 -> OCRedux/2
  IN_DCBusCurrent_A/1 -> OCRedux/1
  OCRedux/1 -> Max/1

== system TorqueCommand/TorqueProfiles ==
  CTRL_VehicleState_en : Inport
  IN_TCDial_na : Inport  Port=2
  Chart : Stateflow chart  TreatAsAtomicUnit=on
  EnumeratedOverMeas : Utilities/EnumeratedOverMeas  sigName='CTRL_TorqueCurve_en'  enumName='TorqueCurve'
  EnumeratedOverMeas1 : Utilities/EnumeratedOverMeas  sigName='CTRL_TCEnable_en'  enumName='TCEnable'
  EnumeratedOverMeas2 : Utilities/EnumeratedOverMeas  sigName='CTRL_TorqueProfile_en'  enumName='TorqueProfile'
  EnumeratedOverMeas3 : Utilities/EnumeratedOverMeas  sigName='CTRL_RegenEnable_en'  enumName='RegenEnable'
  OverMeas : Utilities/OverMeas  sigName='CTRL_TCSensitivity_na'  minimum=-inf  maximum=inf
  CTRL_TorqueCurve_en : Outport
  CTRL_TCSensitivity_int : Outport  Port=2
  CTRL_TorqueProfile_en : Outport  Port=3
  CTRL_TCEnable_en : Outport  Port=4
  CTRL_RegenEnable_en : Outport  Port=5
  wires:
  EnumeratedOverMeas1/1 -> CTRL_TCEnable_en/1  "CTRL_TCEnable_en"
  EnumeratedOverMeas3/1 -> CTRL_RegenEnable_en/1  "CTRL_RegenEnable_en"
  Chart/5(TC) -> EnumeratedOverMeas1/1
  Chart/4(Regen) -> EnumeratedOverMeas3/1
  Chart/2(Curve) -> EnumeratedOverMeas/1
  Chart/1(Profile) -> EnumeratedOverMeas2/1
  CTRL_VehicleState_en/1 -> Chart/2(State)
  EnumeratedOverMeas2/1 -> CTRL_TorqueProfile_en/1  "CTRL_TorqueProfile_en"
  IN_TCDial_na/1 -> Chart/1(TCDial)
  Chart/3(Sensitivity) -> OverMeas/1
  OverMeas/1 -> CTRL_TCSensitivity_int/1  "CTRL_TCSensitivity_na"
  EnumeratedOverMeas/1 -> CTRL_TorqueCurve_en/1  "CTRL_TorqueCurve_en"

== system TorqueCommand/TractionControl ==
  In1 : Inport
  Out1 : Outport
  wires:
  In1/1 -> Out1/1

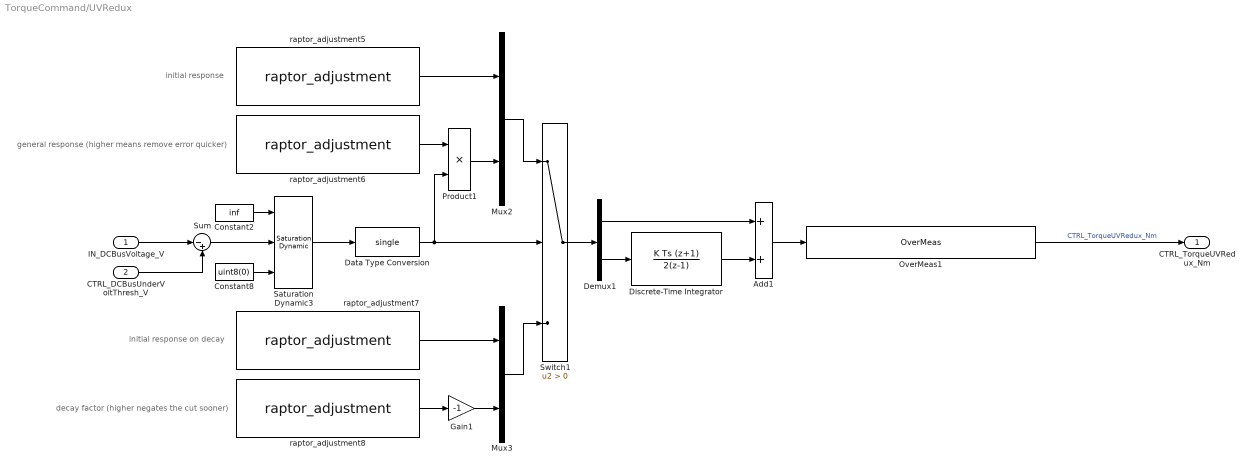
== system TorqueCommand/UVRedux ==
  note: general response (higher means remove error quicker)
  note: initial response
  note: initial response on decay
  note: decay factor (higher negates the cut sooner)
  IN_DCBusVoltage_V : Inport
  CTRL_DCBusUnderVoltThresh_V : Inport  Port=2
  Add1 : Sum
  Constant2 : Constant  Value=inf
  Constant8 : Constant  Value=uint8(0)
  Data Type Conversion : DataTypeConversion  OutDataTypeStr=single  SaturateOnIntegerOverflow=off  RndMeth=Floor
  Demux1 : Demux  Outputs=2
  Discrete-Time Integrator : DiscreteIntegrator  IntegratorMethod=Integration: Trapezoidal  SampleTime=-1  LimitOutput=on  UpperSaturationLimit=TorqueKiUpperSat  LowerSaturationLimit=TorqueKiLowerSat  ICPrevOutput=DiscIntNeverNeededParam  ICPrevScaledInput=DiscIntNeverNeededParam
  Gain1 : Gain  Gain=-1
  Mux2 : Mux  Inputs=2
  Mux3 : Mux  Inputs=2
  OverMeas1 : Utilities/OverMeas  sigName='CTRL_TorqueUVRedux_Nm'  minimum=-inf  maximum=inf
  Product1 : Product
  Saturation Dynamic3 : simulink/Discontinuities/Saturation Dynamic  OutMin=[]  OutMax=[]  OutDataTypeStr=Inherit: Same as second input  OutDataType=fixdt(1, 16)  OutScaling=2^-10  DoSatur=off
  Sum : Sum  Inputs=|-+
  Switch1 : Switch  Criteria=u2 > Threshold  SaturateOnIntegerOverflow=off  InputSameDT=off
  raptor_adjustment5 : Raptor_lib/Data Storage/raptor_adjustment  paramName='CTRL_VoltKpLim_na'  nameSource=Parameter  initValue=10  dataType=single  storage=Calibration  calDispType=Number  calEnum={'False', 'True'}  calGain=1.0  calOffset=0.0  calMax=inf  calMin=-inf  calFormat='-1'  calUnit=''  calHelp=''  calAccess=1  calFunction=raptor_xcp_function(gcb)  calDispHeaders=off  calColHeaders={'Col1' 'Col2' 'Col3'}  calRowHeaders={'Row1' 'Row2' 'Row3'}
      settings: SourceProductName=Raptor
  raptor_adjustment6 : Raptor_lib/Data Storage/raptor_adjustment  paramName='CTRL_VoltKiLim_na'  nameSource=Parameter  initValue=2  dataType=single  storage=Calibration  calDispType=Number  calEnum={'False', 'True'}  calGain=1.0  calOffset=0.0  calMax=inf  calMin=-inf  calFormat='-1'  calUnit=''  calHelp=''  calAccess=1  calFunction=raptor_xcp_function(gcb)  calDispHeaders=off  calColHeaders={'Col1' 'Col2' 'Col3'}  calRowHeaders={'Row1' 'Row2' 'Row3'}
      settings: SourceProductName=Raptor
  raptor_adjustment7 : Raptor_lib/Data Storage/raptor_adjustment  paramName='CTRL_VoltKpLimDecay_na'  nameSource=Parameter  initValue=0  dataType=single  storage=Calibration  calDispType=Number  calEnum={'False', 'True'}  calGain=1.0  calOffset=0.0  calMax=inf  calMin=-inf  calFormat='-1'  calUnit=''  calHelp=''  calAccess=1  calFunction=raptor_xcp_function(gcb)  calDispHeaders=off  calColHeaders={'Col1' 'Col2' 'Col3'}  calRowHeaders={'Row1' 'Row2' 'Row3'}
      settings: SourceProductName=Raptor
  raptor_adjustment8 : Raptor_lib/Data Storage/raptor_adjustment  paramName='CTRL_VoltKiLimDecay_na'  nameSource=Parameter  initValue=250  dataType=single  storage=Calibration  calDispType=Number  calEnum={'False', 'True'}  calGain=1.0  calOffset=0.0  calMax=inf  calMin=-inf  calFormat='-1'  calUnit=''  calHelp=''  calAccess=1  calFunction=raptor_xcp_function(gcb)  calDispHeaders=off  calColHeaders={'Col1' 'Col2' 'Col3'}  calRowHeaders={'Row1' 'Row2' 'Row3'}
      settings: SourceProductName=Raptor
  CTRL_TorqueUVRedux_Nm : Outport
  wires:
  Saturation Dynamic3/1 -> Data Type Conversion/1
  IN_DCBusVoltage_V/1 -> Sum/1
  CTRL_DCBusUnderVoltThresh_V/1 -> Sum/2
  OverMeas1/1 -> CTRL_TorqueUVRedux_Nm/1  "CTRL_TorqueUVRedux_Nm"
  raptor_adjustment6/1 -> Product1/1
  Switch1/1 -> Demux1/1
  Add1/1 -> OverMeas1/1
  Constant8/1 -> Saturation Dynamic3/3
  Product1/1 -> Mux2/2
  Data Type Conversion/1 -> Switch1/2, Product1/2
  Mux2/1 -> Switch1/1
  Gain1/1 -> Mux3/2
  Constant2/1 -> Saturation Dynamic3/1
  Sum/1 -> Saturation Dynamic3/2
  raptor_adjustment5/1 -> Mux2/1
  Demux1/2 -> Discrete-Time Integrator/1
  Mux3/1 -> Switch1/3
  raptor_adjustment7/1 -> Mux3/1
  Discrete-Time Integrator/1 -> Add1/2
  Demux1/1 -> Add1/1
  raptor_adjustment8/1 -> Gain1/1

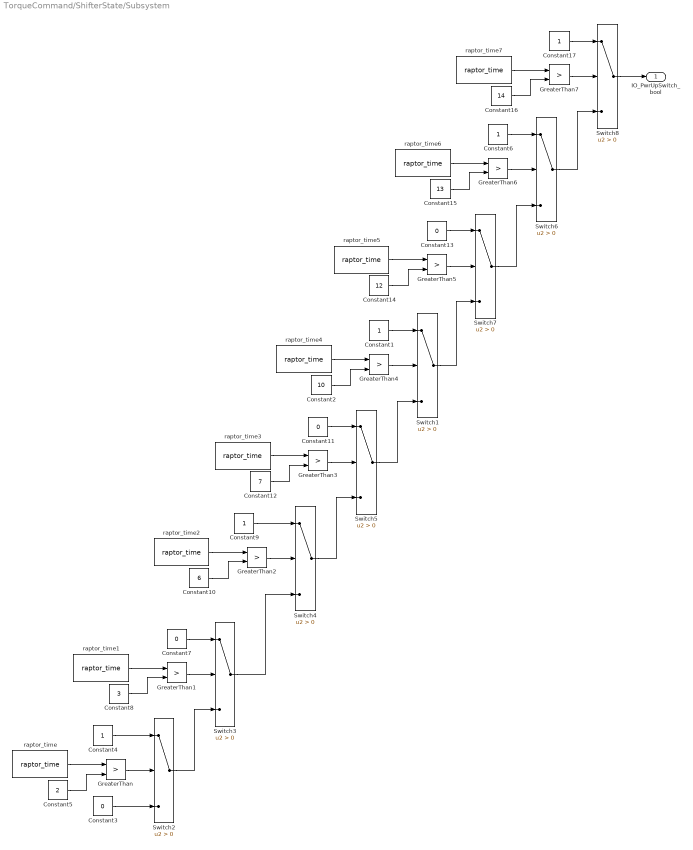
== system TorqueCommand/ShifterState/Subsystem ==
  Constant{1,4,6,9,17} (5 alike) : Constant
  Constant10 : Constant  Value=6
  Constant{3,7,11,13} (4 alike) : Constant  Value=0
  Constant12 : Constant  Value=7
  Constant14 : Constant  Value=12
  Constant15 : Constant  Value=13
  Constant16 : Constant  Value=14
  Constant2 : Constant  Value=10
  Constant5 : Constant  Value=2
  Constant8 : Constant  Value=3
  GreaterThan{,1..7} (8 alike) : RelationalOperator  Operator=>  OutDataTypeStr=boolean  RndMeth=Simplest  InputSameDT=off
  Switch{1..8} (8 alike) : Switch  Criteria=u2 > Threshold  SaturateOnIntegerOverflow=off  InputSameDT=off
  raptor_time{,1..7} (8 alike) : Raptor_lib/Triggers/raptor_time  unit=seconds
      settings: SourceProductName=Raptor
  IO_PwrUpSwitch_bool : Outport
  wires:
  Switch8/1 -> IO_PwrUpSwitch_bool/1
  GreaterThan7/1 -> Switch8/2
  Switch6/1 -> Switch8/3
  Constant16/1 -> GreaterThan7/2
  Constant17/1 -> Switch8/1
  raptor_time7/1 -> GreaterThan7/1
  Switch1/1 -> Switch7/3
  Constant14/1 -> GreaterThan5/2
  Constant15/1 -> GreaterThan6/2
  raptor_time5/1 -> GreaterThan5/1
  Constant6/1 -> Switch6/1
  GreaterThan5/1 -> Switch7/2
  GreaterThan6/1 -> Switch6/2
  raptor_time6/1 -> GreaterThan6/1
  Switch7/1 -> Switch6/3
  Constant13/1 -> Switch7/1
  Constant2/1 -> GreaterThan4/2
  Switch5/1 -> Switch1/3
  raptor_time4/1 -> GreaterThan4/1
  GreaterThan4/1 -> Switch1/2
  Constant1/1 -> Switch1/1
  Constant11/1 -> Switch5/1
  Constant8/1 -> GreaterThan1/2
  raptor_time1/1 -> GreaterThan1/1
  GreaterThan1/1 -> Switch3/2
  Switch4/1 -> Switch5/3
  GreaterThan3/1 -> Switch5/2
  raptor_time3/1 -> GreaterThan3/1
  raptor_time2/1 -> GreaterThan2/1
  Switch3/1 -> Switch4/3
  Constant10/1 -> GreaterThan2/2
  raptor_time/1 -> GreaterThan/1
  GreaterThan/1 -> Switch2/2
  Constant9/1 -> Switch4/1
  Constant5/1 -> GreaterThan/2
  Constant7/1 -> Switch3/1
  Constant3/1 -> Switch2/3
  Constant4/1 -> Switch2/1
  Switch2/1 -> Switch3/3
  Constant12/1 -> GreaterThan3/2
  GreaterThan2/1 -> Switch4/2

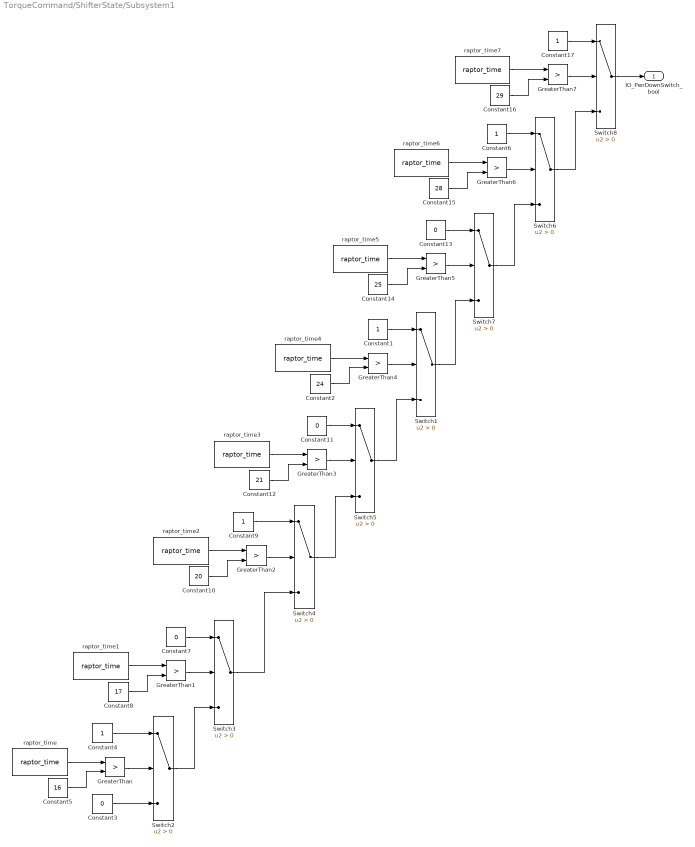
== system TorqueCommand/ShifterState/Subsystem1 ==
  Constant{1,4,6,9,17} (5 alike) : Constant
  Constant10 : Constant  Value=20
  Constant{3,7,11,13} (4 alike) : Constant  Value=0
  Constant12 : Constant  Value=21
  Constant14 : Constant  Value=25
  Constant15 : Constant  Value=28
  Constant16 : Constant  Value=29
  Constant2 : Constant  Value=24
  Constant5 : Constant  Value=16
  Constant8 : Constant  Value=17
  GreaterThan{,1..7} (8 alike) : RelationalOperator  Operator=>  OutDataTypeStr=boolean  RndMeth=Simplest  InputSameDT=off
  Switch{1..8} (8 alike) : Switch  Criteria=u2 > Threshold  SaturateOnIntegerOverflow=off  InputSameDT=off
  raptor_time{,1..7} (8 alike) : Raptor_lib/Triggers/raptor_time  unit=seconds
      settings: SourceProductName=Raptor
  IO_PwrDownSwitch_bool : Outport
  wires:
  Switch8/1 -> IO_PwrDownSwitch_bool/1
  GreaterThan7/1 -> Switch8/2
  Switch6/1 -> Switch8/3
  Constant16/1 -> GreaterThan7/2
  Constant17/1 -> Switch8/1
  raptor_time7/1 -> GreaterThan7/1
  Switch1/1 -> Switch7/3
  Constant14/1 -> GreaterThan5/2
  Constant15/1 -> GreaterThan6/2
  raptor_time5/1 -> GreaterThan5/1
  Constant6/1 -> Switch6/1
  GreaterThan5/1 -> Switch7/2
  GreaterThan6/1 -> Switch6/2
  raptor_time6/1 -> GreaterThan6/1
  Switch7/1 -> Switch6/3
  Constant13/1 -> Switch7/1
  Constant2/1 -> GreaterThan4/2
  Switch5/1 -> Switch1/3
  raptor_time4/1 -> GreaterThan4/1
  GreaterThan4/1 -> Switch1/2
  Constant1/1 -> Switch1/1
  Constant11/1 -> Switch5/1
  Constant8/1 -> GreaterThan1/2
  raptor_time1/1 -> GreaterThan1/1
  GreaterThan1/1 -> Switch3/2
  Switch4/1 -> Switch5/3
  GreaterThan3/1 -> Switch5/2
  raptor_time3/1 -> GreaterThan3/1
  raptor_time2/1 -> GreaterThan2/1
  Switch3/1 -> Switch4/3
  Constant10/1 -> GreaterThan2/2
  raptor_time/1 -> GreaterThan/1
  GreaterThan/1 -> Switch2/2
  Constant9/1 -> Switch4/1
  Constant5/1 -> GreaterThan/2
  Constant7/1 -> Switch3/1
  Constant3/1 -> Switch2/3
  Constant4/1 -> Switch2/1
  Switch2/1 -> Switch3/3
  Constant12/1 -> GreaterThan3/2
  GreaterThan2/1 -> Switch4/2

== system TorqueCommand/TorqueCommand/Subsystem2 ==
  note: decrease at 150A
  note: decrease at 180A
  note: decrease at 180A
  IN_DCBusCurrent_A : Inport
  CTRL_CurrentTorqueSetting_na : Inport  Port=2
  Multiport Switch : MultiPortSwitch  SaturateOnIntegerOverflow=off  InputSameDT=off
  raptor_table_1d1 : Raptor_lib/Table Lookup/raptor_table_1d  dataName='CTRL_CurrentToLimTorqueCmd2_1D'  initValue=[230;230;226;214;194;166;130;86;34;0]  dataType=single  storage=Calibration  initValueX=[0;180;190;200;210;220;230;240;250;260]  dataTypeXY=single  storageXY=Calibration  calVisible=on  showTable=on  calGain=1.0  calOffset=0.0  calMax=Inf  calMin=-Inf  calFormat='-1'  calUnit='Nm'  calHelp=''  showBreakpoint=on  dataNameX=[]  calGainX=1.0  calOffsetX=0.0  calMaxX=Inf  calMinX=-Inf  calFormatX='-1'  calUnitX='A'  calHelpX=''  calAccess=1  calFunction=raptor_xcp_function(gcb)  measureEnable=off  mName=['Data1D_Output']
      settings: SourceProductName=Raptor
  raptor_table_1d2 : Raptor_lib/Table Lookup/raptor_table_1d  dataName='CTRL_CurrentToLimTorqueCmd_1D'  initValue=[230;228;226;222;218;212;206;198;190;180;170;158;146;132;118;102;86;68;50;30;10;0]  dataType=single  storage=Calibration  initValueX=[0;150;155;160;165;170;175;180;185;190;195;200;205;210;215;220;225;230;235;240;245;250]  dataTypeXY=single  storageXY=Calibration  calVisible=on  showTable=on  calGain=1.0  calOffset=0.0  calMax=Inf  calMin=-Inf  calFormat='-1'  calUnit='Nm'  calHelp=''  showBreakpoint=on  dataNameX=[]  calGainX=1.0  calOffsetX=0.0  calMaxX=Inf  calMinX=-Inf  calFormatX='-1'  calUnitX='A'  calHelpX=''  calAccess=1  calFunction=raptor_xcp_function(gcb)  measureEnable=off  mName=['Data1D_Output']
      settings: SourceProductName=Raptor
  raptor_table_1d3 : Raptor_lib/Table Lookup/raptor_table_1d  dataName='CTRL_CurrentToLimTorqueCmd3_1D'  initValue=[230;230;226;214;194;166;130;86;34;0]  dataType=single  storage=Calibration  initValueX=[0;150;160;170;180;190;200;210;220;230]  dataTypeXY=single  storageXY=Calibration  calVisible=on  showTable=on  calGain=1.0  calOffset=0.0  calMax=Inf  calMin=-Inf  calFormat='-1'  calUnit='Nm'  calHelp=''  showBreakpoint=on  dataNameX=[]  calGainX=1.0  calOffsetX=0.0  calMaxX=Inf  calMinX=-Inf  calFormatX='-1'  calUnitX='A'  calHelpX=''  calAccess=1  calFunction=raptor_xcp_function(gcb)  measureEnable=off  mName=['Data1D_Output']
      settings: SourceProductName=Raptor
  CTRL_CurrentTorqueLimit_Nm : Outport
  wires:
  Multiport Switch/1 -> CTRL_CurrentTorqueLimit_Nm/1
  IN_DCBusCurrent_A/1 -> raptor_table_1d2/1, raptor_table_1d1/1, raptor_table_1d3/1
  raptor_table_1d3/1 -> Multiport Switch/4
  raptor_table_1d1/1 -> Multiport Switch/3
  raptor_table_1d2/1 -> Multiport Switch/2
  CTRL_CurrentTorqueSetting_na/1 -> Multiport Switch/1

== system TorqueCommand/TorqueCommand/Subsystem3 ==
  IN_DCBusVoltage_V : Inport
  CTRL_VoltageTorqueSetting_na : Inport  Port=2
  Multiport Switch : MultiPortSwitch  SaturateOnIntegerOverflow=off  InputSameDT=off
  raptor_table_1d1 : Raptor_lib/Table Lookup/raptor_table_1d  dataName='CTRL_VoltageToLimTorqueCmd2_1D'  initValue=[0;0;230;230]  dataType=double  storage=Calibration  initValueX=[0;225;280;378]  dataTypeXY=double  storageXY=Calibration  calVisible=on  showTable=on  calGain=1.0  calOffset=0.0  calMax=Inf  calMin=-Inf  calFormat='-1'  calUnit='Nm'  calHelp=''  showBreakpoint=on  dataNameX=[]  calGainX=1.0  calOffsetX=0.0  calMaxX=Inf  calMinX=-Inf  calFormatX='-1'  calUnitX='V'  calHelpX=''  calAccess=1  calFunction=raptor_xcp_function(gcb)  measureEnable=off  mName=['Data1D_Output']
      settings: SourceProductName=Raptor
  raptor_table_1d2 : Raptor_lib/Table Lookup/raptor_table_1d  dataName='CTRL_VoltageToLimTorqueCmd_1D'  initValue=[0;0;230;230]  dataType=double  storage=Calibration  initValueX=[0;225;280;378]  dataTypeXY=double  storageXY=Calibration  calVisible=on  showTable=on  calGain=1.0  calOffset=0.0  calMax=Inf  calMin=-Inf  calFormat='-1'  calUnit='Nm'  calHelp=''  showBreakpoint=on  dataNameX=[]  calGainX=1.0  calOffsetX=0.0  calMaxX=Inf  calMinX=-Inf  calFormatX='-1'  calUnitX='V'  calHelpX=''  calAccess=1  calFunction=raptor_xcp_function(gcb)  measureEnable=off  mName=['Data1D_Output']
      settings: SourceProductName=Raptor
  raptor_table_1d3 : Raptor_lib/Table Lookup/raptor_table_1d  dataName='CTRL_VoltageToLimTorqueCmd3_1D'  initValue=[0;0;230;230]  dataType=double  storage=Calibration  initValueX=[0;225;280;378]  dataTypeXY=double  storageXY=Calibration  calVisible=on  showTable=on  calGain=1.0  calOffset=0.0  calMax=Inf  calMin=-Inf  calFormat='-1'  calUnit='Nm'  calHelp=''  showBreakpoint=on  dataNameX=[]  calGainX=1.0  calOffsetX=0.0  calMaxX=Inf  calMinX=-Inf  calFormatX='-1'  calUnitX='V'  calHelpX=''  calAccess=1  calFunction=raptor_xcp_function(gcb)  measureEnable=off  mName=['Data1D_Output']
      settings: SourceProductName=Raptor
  CTRL_CurrentTorqueLimit_Nm : Outport
  wires:
  CTRL_VoltageTorqueSetting_na/1 -> Multiport Switch/1
  raptor_table_1d2/1 -> Multiport Switch/2
  raptor_table_1d1/1 -> Multiport Switch/3
  raptor_table_1d3/1 -> Multiport Switch/4
  IN_DCBusVoltage_V/1 -> raptor_table_1d1/1, raptor_table_1d3/1, raptor_table_1d2/1
  Multiport Switch/1 -> CTRL_CurrentTorqueLimit_Nm/1

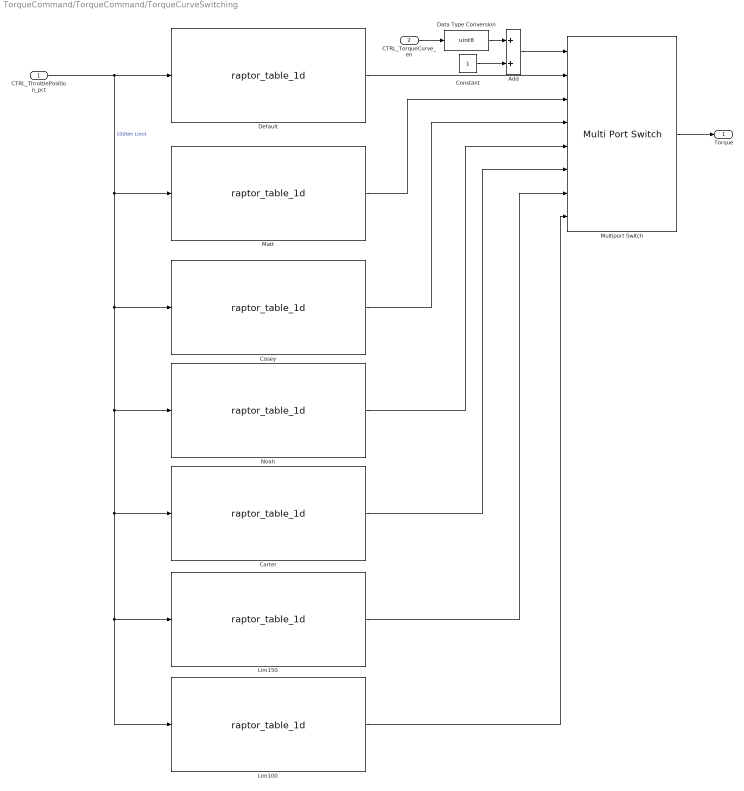
== system TorqueCommand/TorqueCommand/TorqueCurveSwitching ==
  CTRL_ThrottlePosition_pct : Inport
  CTRL_TorqueCurve_en : Inport  Port=2
  Add : Sum
  Carter : Raptor_lib/Table Lookup/raptor_table_1d  dataName='CTRL_ThrottleToTorqueCmdCarter_1D'  initValue=[0;1;3;6;11;18;25;34;45;57;70;85;101;118;137;158;179;202;227;230;230]  dataType=single  storage=Calibration  initValueX=[0;5;10;15;20;25;30;35;40;45;50;55;60;65;70;75;80;85;90;95;100]  dataTypeXY=single  storageXY=Calibration  calVisible=on  showTable=on  calGain=1.0  calOffset=0.0  calMax=Inf  calMin=-Inf  calFormat='-1'  calUnit='pct'  calHelp=''  showBreakpoint=on  dataNameX=[]  calGainX=1.0  calOffsetX=0.0  calMaxX=Inf  calMinX=-Inf  calFormatX='-1'  calUnitX='Nm'  calHelpX=''  calAccess=1  calFunction=raptor_xcp_function(gcb)  measureEnable=off  mName=['Data1D_Output']
      settings: SourceProductName=Raptor
  Casey : Raptor_lib/Table Lookup/raptor_table_1d  dataName='CTRL_ThrottleToTorqueCmdCasey_1D'  initValue=[0;3;6;9;12;15;25;35;45;55;65;75;85;95;105;115;135;155;175;195;200]  dataType=single  storage=Calibration  initValueX=[0;5;10;15;20;25;30;35;40;45;50;55;60;65;70;75;80;85;90;95;100]  dataTypeXY=single  storageXY=Calibration  calVisible=on  showTable=on  calGain=1.0  calOffset=0.0  calMax=Inf  calMin=-Inf  calFormat='-1'  calUnit='pct'  calHelp=''  showBreakpoint=on  dataNameX=[]  calGainX=1.0  calOffsetX=0.0  calMaxX=Inf  calMinX=-Inf  calFormatX='-1'  calUnitX='Nm'  calHelpX=''  calAccess=1  calFunction=raptor_xcp_function(gcb)  measureEnable=off  mName=['Data1D_Output']
      settings: SourceProductName=Raptor
  Constant : Constant
  Data Type Conversion : DataTypeConversion  OutDataTypeStr=uint8  SaturateOnIntegerOverflow=off  RndMeth=Floor
  Default : Raptor_lib/Table Lookup/raptor_table_1d  dataName='CTRL_ThrottleToTorqueCmdDef_1D'  initValue=[0;3;6;9;12;15;25;35;45;55;65;75;85;95;105;115;135;155;175;195;200]  dataType=single  storage=Calibration  initValueX=[0;5;10;15;20;25;30;35;40;45;50;55;60;65;70;75;80;85;90;95;100]  dataTypeXY=single  storageXY=Calibration  calVisible=on  showTable=on  calGain=1.0  calOffset=0.0  calMax=Inf  calMin=-Inf  calFormat='-1'  calUnit='pct'  calHelp=''  showBreakpoint=on  dataNameX=[]  calGainX=1.0  calOffsetX=0.0  calMaxX=Inf  calMinX=-Inf  calFormatX='-1'  calUnitX='Nm'  calHelpX=''  calAccess=1  calFunction=raptor_xcp_function(gcb)  measureEnable=off  mName=['Data1D_Output']
      settings: SourceProductName=Raptor
  Lim100 : Raptor_lib/Table Lookup/raptor_table_1d  dataName='CTRL_ThrottleToTorqueCmd100_1D'  initValue=[0;8;17;25;33;40;48;55;62;68;74;79;84;88;92;95;97;99;100;100;100]  dataType=single  storage=Calibration  initValueX=[0;5;10;15;20;25;30;35;40;45;50;55;60;65;70;75;80;85;90;95;100]  dataTypeXY=single  storageXY=Calibration  calVisible=on  showTable=on  calGain=1.0  calOffset=0.0  calMax=Inf  calMin=-Inf  calFormat='-1'  calUnit='pct'  calHelp=''  showBreakpoint=on  dataNameX=[]  calGainX=1.0  calOffsetX=0.0  calMaxX=Inf  calMinX=-Inf  calFormatX='-1'  calUnitX='Nm'  calHelpX=''  calAccess=1  calFunction=raptor_xcp_function(gcb)  measureEnable=off  mName=['Data1D_Output']
      settings: SourceProductName=Raptor
  Lim150 : Raptor_lib/Table Lookup/raptor_table_1d  dataName='CTRL_ThrottleToTorqueCmd150_1D'  initValue=[0;8;17;25;33;40;48;55;62;68;74;79;84;88;92;95;97;99;100;100;100]  dataType=single  storage=Calibration  initValueX=[0;5;10;15;20;25;30;35;40;45;50;55;60;65;70;75;80;85;90;95;100]  dataTypeXY=single  storageXY=Calibration  calVisible=on  showTable=on  calGain=1.0  calOffset=0.0  calMax=Inf  calMin=-Inf  calFormat='-1'  calUnit='pct'  calHelp=''  showBreakpoint=on  dataNameX=[]  calGainX=1.0  calOffsetX=0.0  calMaxX=Inf  calMinX=-Inf  calFormatX='-1'  calUnitX='Nm'  calHelpX=''  calAccess=1  calFunction=raptor_xcp_function(gcb)  measureEnable=off  mName=['Data1D_Output']
      settings: SourceProductName=Raptor
  Matt : Raptor_lib/Table Lookup/raptor_table_1d  dataName='CTRL_ThrottleToTorqueCmdMatt_1D'  initValue=[0;3;6;9;12;15;25;35;45;55;65;75;85;95;105;115;135;155;175;195;200]  dataType=single  storage=Calibration  initValueX=[0;5;10;15;20;25;30;35;40;45;50;55;60;65;70;75;80;85;90;95;100]  dataTypeXY=single  storageXY=Calibration  calVisible=on  showTable=on  calGain=1.0  calOffset=0.0  calMax=Inf  calMin=-Inf  calFormat='-1'  calUnit='pct'  calHelp=''  showBreakpoint=on  dataNameX=[]  calGainX=1.0  calOffsetX=0.0  calMaxX=Inf  calMinX=-Inf  calFormatX='-1'  calUnitX='Nm'  calHelpX=''  calAccess=1  calFunction=raptor_xcp_function(gcb)  measureEnable=off  mName=['Data1D_Output']
      settings: SourceProductName=Raptor
  Multiport Switch : MultiPortSwitch  Inputs=7  SaturateOnIntegerOverflow=off  InputSameDT=off
  Noah : Raptor_lib/Table Lookup/raptor_table_1d  dataName='CTRL_ThrottleToTorqueCmdNoah_1D'  initValue=[0;3;6;9;12;15;25;35;45;55;65;75;85;95;105;115;135;155;175;195;200]  dataType=single  storage=Calibration  initValueX=[0;5;10;15;20;25;30;35;40;45;50;55;60;65;70;75;80;85;90;95;100]  dataTypeXY=single  storageXY=Calibration  calVisible=on  showTable=on  calGain=1.0  calOffset=0.0  calMax=Inf  calMin=-Inf  calFormat='-1'  calUnit='pct'  calHelp=''  showBreakpoint=on  dataNameX=[]  calGainX=1.0  calOffsetX=0.0  calMaxX=Inf  calMinX=-Inf  calFormatX='-1'  calUnitX='Nm'  calHelpX=''  calAccess=1  calFunction=raptor_xcp_function(gcb)  measureEnable=off  mName=['Data1D_Output']
      settings: SourceProductName=Raptor
  Torque : Outport
  wires:
  CTRL_ThrottlePosition_pct/1 -> Default/1, Lim150/1, Lim100/1, Carter/1, Noah/1, Casey/1, Matt/1  "100Nm Limit"
  Default/1 -> Multiport Switch/2
  Matt/1 -> Multiport Switch/3
  Casey/1 -> Multiport Switch/4
  Noah/1 -> Multiport Switch/5
  Carter/1 -> Multiport Switch/6
  Lim150/1 -> Multiport Switch/7
  Lim100/1 -> Multiport Switch/8
  Multiport Switch/1 -> Torque/1
  CTRL_TorqueCurve_en/1 -> Data Type Conversion/1
  Add/1 -> Multiport Switch/1
  Constant/1 -> Add/2
  Data Type Conversion/1 -> Add/1
